simulink model "rev_testUDPethernetShield"  (R2019b)
settings: Solver=FixedStepAuto  StartTime=0.0  StopTime=inf  FixedStep=0.1  RelTol=1e-3
undefined symbols (not defined in the file): f
libraries: xpcutilitieslib x1, instrumentlib x1
settings Model: Creator=ONLY-GOD  LastModifiedBy=ONLY-GOD

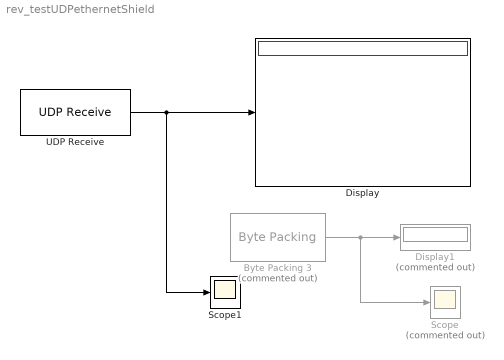
== system rev_testUDPethernetShield ==
  Byte Packing 3 : xpcutilitieslib/Byte Packing   Commented=on  MaskPackedDataType=single  MaskUnpackedDataTypes={'uint8'}  MaskAlignment=4
  Display : Display
  Display1 : Display  Commented=on
  Scope : Scope  Commented=on
  Scope1 : Scope
  UDP Receive : instrumentlib/UDP Receive  Host=192.168.0.252  Port=50002  LocalPort=50001  EnablePortSharing=off  GetLatestData=off  DataSize=1  DataType=uint8  ASCIIFormatting=%f,  Terminator=LF  ByteOrder=BigEndian  EnableBlockingMode=on  Timeout=10  SampleTime=0.1  LocalAddress=192.168.0.116
      settings: SourceProductName=Instrument Control Toolbox
  wires:
  Byte Packing 3/1 -> Scope/1, Display1/1
  UDP Receive/1 -> Scope1/1, Display/1
